simulink model "LookupTableND_2D_1"  (R2017b)
settings: Solver=FixedStepDiscrete  StartTime=0.0  StopTime=10.0  FixedStep=0.200000  RelTol=1e-3  EnableMultiTasking=on
model workspace (MAT data in the model file):
  compositionalMap.analysisNames = {'n_minus_DLookupTable_40_011_ext_node'}
  compositionalMap.compositionalOptions = {{''}}
  compositionalMap.selectedOptions = 1
  nodeNameToBlockNameMap = containers.Map
  nodeNameToBlockNameMap.serialization.keys = {'In1_1', 'In2_1', 'LookupTableND_2D_1_PP', 'Out1_1', 'n_minus_DLookupTable_1'}
  nodeNameToBlockNameMap.serialization.values{1} = 'LookupTableND_2D_1_PP/In1'
  nodeNameToBlockNameMap.serialization.values{2} = 'LookupTableND_2D_1_PP/In2'
  nodeNameToBlockNameMap.serialization.values{3} = 'LookupTableND_2D_1_PP'
  nodeNameToBlockNameMap.serialization.values{4} = 'LookupTableND_2D_1_PP/Out1'
  nodeNameToBlockNameMap.serialization.values{5} = 'LookupTableND_2D_1_PP/n-D Lookup
    | Table'
  nodeNameToBlockNameMap.serialization.uniformity = 1
  nodeNameToBlockNameMap.serialization.keyType = 'char'
  nodeNameToBlockNameMap.serialization.valueType = 'char'
  verificationResults.analysisResults{1}.top = 'n_minus_DLookupTable_40_011_ext_node'
  verificationResults.analysisResults{1}.abstract = ''
  verificationResults.analysisResults{1}.concrete = ''
  verificationResults.analysisResults{1}.assumptions = ''
  verificationResults.analysisResults{1}.properties = {}
  verificationResults.sampleTime = 0.2
settings Model: Creator=hbourbou  LastModifiedBy=hbourbou
settings DataIOCC: LimitDataPoints=on  SaveFormat=StructureWithTime
settings OptimizationCC: LifeSpan=inf
settings DebuggingCC: SFUnexpectedBacktrackingDiag=warning  SFNoUnconditionalDefaultTransitionDiag=warning  SFExecutionAtInitializationDiag=none
settings HardwareCC: ProdBitPerSizeT=32  ProdBitPerPtrDiffT=32  ProdWordSize=32  ProdHWDeviceType=Specified
settings ModelReferenceCC: PropagateSignalLabelsOutOfModel=off
settings CodeAppCC: StateflowObjectComments=on
settings GRTTargetCC: TargetLangStandard=C89/C90 (ANSI)
settings ConfigComp: CovMetricSettings=dw  CovHtmlReporting=on  CovSaveCumulativeToWorkspaceVar=on  CovSaveSingleToWorkspaceVar=on  CovExternalEMLEnable=off

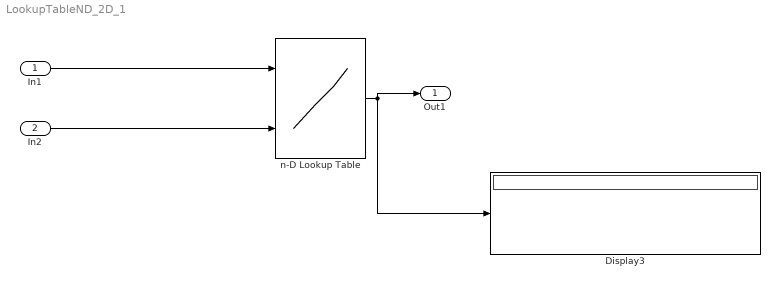
== system LookupTableND_2D_1 ==
  In1 : Inport
  In2 : Inport  Port=2
  Display3 : Display
  n-D Lookup Table : Lookup_n-D  BreakpointsForDimension1=[1.2 2.3 3.9]  BreakpointsForDimension2=[0 1.5 2]  BreakpointsForDimension3=[5 6]  Table=[1 2 3; 4 5 6 ; 7 8 9]  InternalRulePriority=Speed  RndMeth=Simplest  InputSameDT=on
  Out1 : Outport
  wires:
  In1/1 -> n-D Lookup Table/1
  In2/1 -> n-D Lookup Table/2
  n-D Lookup Table/1 -> Out1/1, Display3/1
